simulink model "circuito_RL"  (R2019b)
settings: Solver=VariableStepAuto  StartTime=0.0  StopTime=0.04  RelTol=1e-3
settings Model: Creator=fernandopassold  LastModifiedBy=fernandopassold

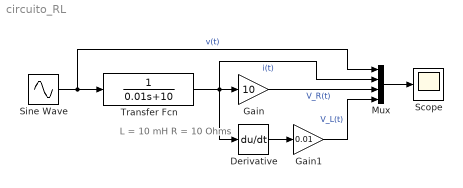
== system circuito_RL ==
  note: L = 10 mH
      | R = 10 Ohms
  Derivative : Derivative
  Gain : Gain  Gain=10
  Gain1 : Gain  Gain=0.01
  Mux : Mux
  Scope : Scope
  Sine Wave : Sin  Frequency=2*pi*100  SampleTime=0
  Transfer Fcn : TransferFcn  Denominator=[0.01 10]
  wires:
  Sine Wave/1 -> Mux/1, Transfer Fcn/1  "v(t)"
  Transfer Fcn/1 -> Derivative/1, Mux/2, Gain/1  "i(t)"
  Gain/1 -> Mux/3  "V_R(t)"
  Mux/1 -> Scope/1
  Derivative/1 -> Gain1/1
  Gain1/1 -> Mux/4  "V_L(t)"
